simulink model "Copy_of_AJKSnowman"  (R2023a)
settings: Solver=FixedStepDiscrete  StartTime=0.0  StopTime=1  FixedStep=0.01  RelTol=1e-3
libraries: simulink x1

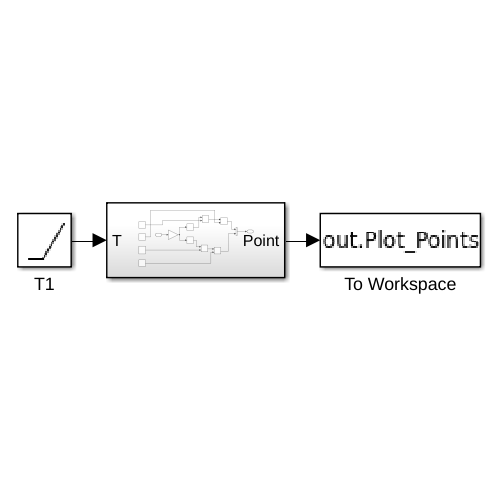
[thumbnail: Simulink's stored preview of the top-level diagram]
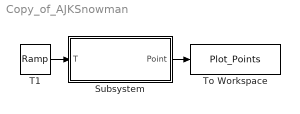
== system Copy_of_AJKSnowman ==
  Subsystem : Subsystem
  T1 : simulink/Sources/Ramp  slope=1  start=0  InitialOutput=0
  To Workspace : ToWorkspace  VariableName=Plot_Points  SampleTime=-1
  wires:
  T1/1 -> Subsystem/1(T)
  Subsystem/1(Point) -> To Workspace/1

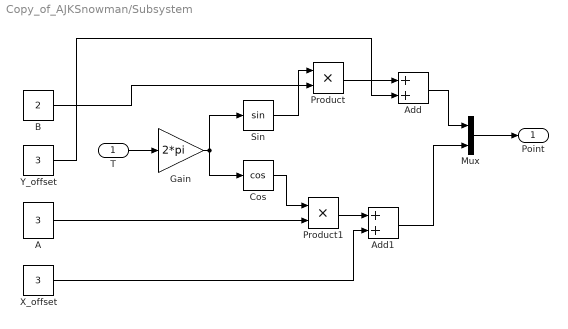
== system Copy_of_AJKSnowman/Subsystem ==
  T : Inport
  A : Constant  Value=3
  Add : Sum
  Add1 : Sum
  B : Constant  Value=2
  Cos : Trigonometry  Operator=cos
  Gain : Gain  Gain=2*pi
  Mux : Mux  Inputs=2
  Product : Product
  Product1 : Product
  Sin : Trigonometry
  X_offset : Constant  Value=3
  Y_offset : Constant  Value=3
  Point : Outport
  wires:
  Y_offset/1 -> Add/2
  Product/1 -> Add/1
  X_offset/1 -> Add1/2
  Add1/1 -> Mux/2
  Cos/1 -> Product1/1
  B/1 -> Product/2
  A/1 -> Product1/2
  Sin/1 -> Product/1
  Gain/1 -> Cos/1, Sin/1
  Product1/1 -> Add1/1
  T/1 -> Gain/1
  Add/1 -> Mux/1
  Mux/1 -> Point/1
